simulink model "bpsk_rec2"  (Simulink 10.1)
settings: Solver=VariableStepAuto  StartTime=0.0  StopTime=1000  RelTol=1e-3
libraries: dsp_blocks x7
settings Model: Creator=rayan  LastModifiedBy=rayan
settings DataIOCC: SaveFormat=Dataset  ReturnWorkspaceOutputs=on
settings OptimizationCC: LifeSpan=auto
settings DebuggingCC: UnderspecifiedInitializationDetection=Simplified  MergeDetectMultiDrivingBlocksExec=error  SFUnexpectedBacktrackingDiag=error  SFNoUnconditionalDefaultTransitionDiag=error  SFExecutionAtInitializationDiag=warning  ArithmeticOperatorsInVariantConditions=error
settings HardwareCC: ProdBitPerPointer=64  ProdBitPerSizeT=64  ProdBitPerPtrDiffT=64  ProdLargestAtomicFloat=Float  ProdIntDivRoundTo=Zero  ProdEndianess=LittleEndian  ProdWordSize=64  ProdHWDeviceType=Intel->x86-64 (Windows64)
settings ModelReferenceCC: PropagateSignalLabelsOutOfModel=on
settings SFSimCC: SimUseLocalCustomCode=on  CustomCodeUndefinedFunction=FilterOut
settings RTWCC: RTWUseLocalCustomCode=on
settings CodeAppCC: StateflowObjectComments=off
settings GRTTargetCC: TargetLangStandard=C99 (ISO)  CombineOutputUpdateFcns=on  GRTInterface=off
settings ConfigComp: CovMetricSettings=dwe  CovHtmlReporting=off  CovSaveCumulativeToWorkspaceVar=off  CovSaveSingleToWorkspaceVar=off  CovExternalEMLEnable=on

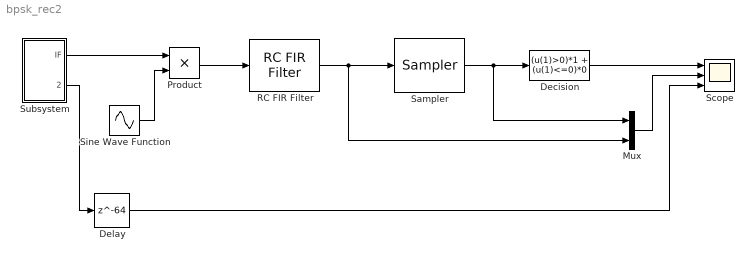
== system bpsk_rec2 ==
  Decision : Fcn  Expr=(u(1)>0)*1 + (u(1)<=0)*0
  Delay : Delay  DelayLength=64
  Mux : Mux  Inputs=2
  Product : Product
  RC FIR Filter : dsp_blocks/Filters/RC FIR Filter  period=50  beta=0.5  root=off  filt_len=128  win_type=on
  Sampler : dsp_blocks/Conversions/Sampler  offset=80  samp_period=50
  Scope : Scope  NumInputPorts=3
  Sine Wave Function : Sin  Amplitude=2  Frequency=2*pi*0.1  SampleTime=0
  Subsystem : Subsystem
  wires:
  Subsystem/1(IF) -> Product/1
  Sine Wave Function/1 -> Product/2
  Subsystem/2(Debug) -> Delay/1
  Product/1 -> RC FIR Filter/1
  RC FIR Filter/1 -> Mux/2, Sampler/1
  Sampler/1 -> Mux/1, Decision/1
  Decision/1 -> Scope/1
  Delay/1 -> Scope/3
  Mux/1 -> Scope/2

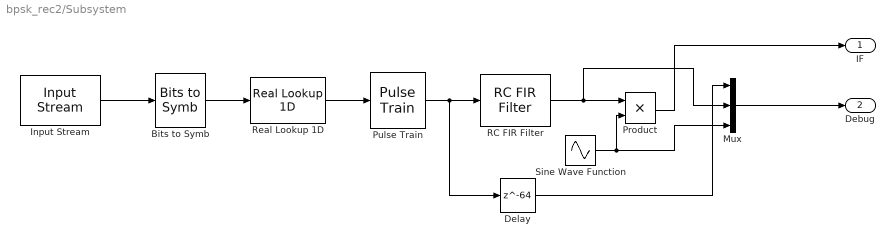
== system bpsk_rec2/Subsystem ==
  Bits to Symb : dsp_blocks/Conversions/Bits to Symb
  Delay : Delay  DelayLength=64
  Input Stream : dsp_blocks/Sources//Sinks/Input Stream  period=50  width=1  fname=rand.mat
  Mux : Mux  Inputs=3
  Product : Product
  Pulse Train : dsp_blocks/Conversions/Pulse Train  period=50
  RC FIR Filter : dsp_blocks/Filters/RC FIR Filter  period=50  beta=0.5  root=off  filt_len=128  win_type=on
  Real Lookup 1D : dsp_blocks/Conversions/Real Lookup 1D  table=[-1 1]
  Sine Wave Function : Sin  Frequency=2*pi*0.1  SampleTime=0
  IF : Outport
  Debug : Outport  Port=2
  wires:
  RC FIR Filter/1 -> Mux/2, Product/1
  Delay/1 -> Mux/1
  Input Stream/1 -> Bits to Symb/1
  Bits to Symb/1 -> Real Lookup 1D/1
  Pulse Train/1 -> Delay/1, RC FIR Filter/1
  Mux/1 -> Debug/1
  Sine Wave Function/1 -> Mux/3, Product/2
  Real Lookup 1D/1 -> Pulse Train/1
  Product/1 -> IF/1
